simulink model "identyfikacja_zawor1_reczny_alfa"  (R2014b)
settings: Solver=ode5  StartTime=0.0  StopTime=40.45  FixedStep=0.05  RelTol=1e-3
values from neighbouring files (symbols this model uses):
  a = 31    [charakterystyka_pompa.m]    (also in charakterystyka_pompa_sterownik.m; dane14listopad.mat; danePompa.mat; pomiary.m)
  alfa = parametry(3)    [wskaznikZawor1alfa.m]
  C1a = parametry(1)    [wskaznikZawor1alfa.m]
  w = 5    [charakterystyka_pompa.m]    (also in charakterystyka_pompa_sterownik.m; dane14listopad.mat; danePompa.mat; pomiary.m)
  x01a = parametry(2)    [wskaznikZawor1alfa.m]
settings Model: Creator=Michal  LastModifiedBy=Michal
settings DebuggingCC: UnderspecifiedInitializationDetection=Classic  MergeDetectMultiDrivingBlocksExec=none

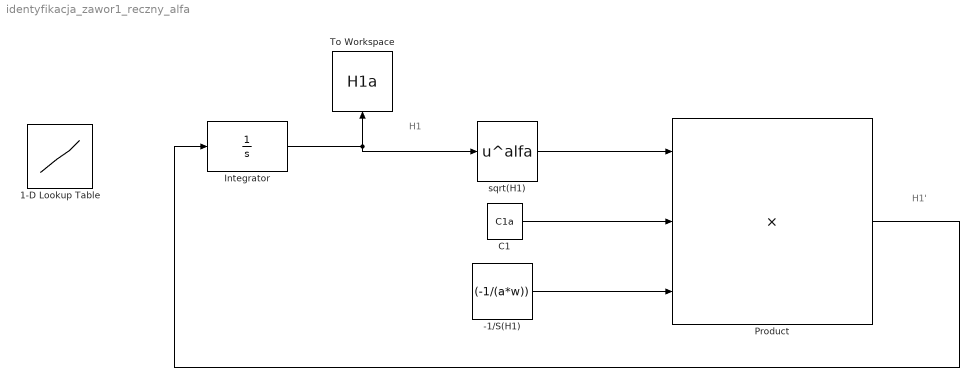
== system identyfikacja_zawor1_reczny_alfa ==
  note: H1'
  note: H1
  -1/S(H1) : Constant  Value=(-1/(a*w))
  1-D Lookup Table : Lookup_n-D  NumberOfTableDimensions=1  BreakpointsForDimension1=[-5:5]  Table=tanh([-5:5])  InternalRulePriority=Speed  RndMeth=Simplest  InputSameDT=on
  "C1 " : Constant  Value=C1a
  Integrator : Integrator  InitialCondition=x01a
  Product : Product  Inputs=3
  To Workspace : ToWorkspace  VariableName=H1a  SaveFormat=Structure With Time  SampleTime=-1
  sqrt(H1) : Fcn  Tag=H1^alfa  Expr=u^alfa
  wires:
  Integrator/1 -> To Workspace/1, sqrt(H1)/1
  sqrt(H1)/1 -> Product/1
  "C1 "/1 -> Product/2
  Product/1 -> Integrator/1
  -1/S(H1)/1 -> Product/3
